simulink model "transfoclarkepark"  (R2018b)
settings: Solver=VariableStepAuto  StartTime=0.0  StopTime=10.0  RelTol=1e-3
settings Model: Creator=lefebvgu  LastModifiedBy=poteaum

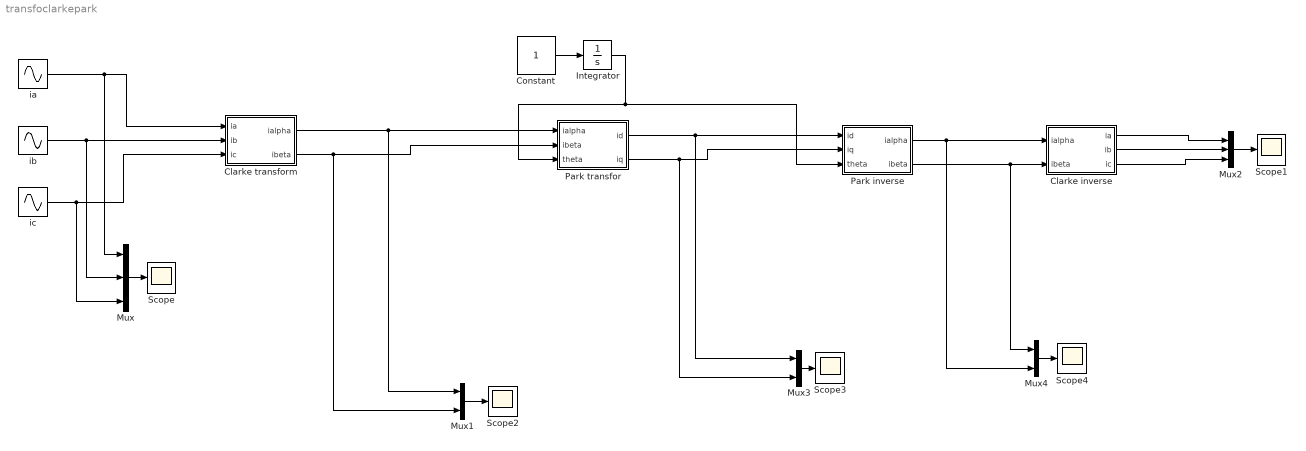
== system transfoclarkepark ==
  Clarke inverse : MATLAB Function  TreatAsAtomicUnit=on
  "Clarke transform " : MATLAB Function  TreatAsAtomicUnit=on
  Constant : Constant  VectorParams1D=off  SampleTime=-1
  Integrator : Integrator
  Mux : Mux  Inputs=3
  Mux1 : Mux  Inputs=2
  Mux2 : Mux  Inputs=3
  Mux3 : Mux  Inputs=2
  Mux4 : Mux  Inputs=2
  "Park inverse " : MATLAB Function  TreatAsAtomicUnit=on
  "Park transfor " : MATLAB Function  TreatAsAtomicUnit=on
  Scope{,1..4} (5 alike) : Scope
  ia : Sin  Amplitude=36  SampleTime=0
  ib : Sin  Amplitude=36  Phase=-2*pi/3  SampleTime=0
  ic : Sin  Amplitude=36  Phase=2*pi/3  SampleTime=0
  wires:
  ia/1 -> Mux/1, "Clarke transform "/1(ia)
  ib/1 -> Mux/2, "Clarke transform "/2(ib)
  ic/1 -> Mux/3, "Clarke transform "/3(ic)
  Mux/1 -> Scope/1
  Clarke inverse/1(ia) -> Mux2/1
  Clarke inverse/2(ib) -> Mux2/2
  Clarke inverse/3(ic) -> Mux2/3
  Mux2/1 -> Scope1/1
  "Clarke transform "/1(ialpha) -> Mux1/1, "Park transfor "/1(ialpha)
  "Clarke transform "/2(ibeta) -> Mux1/2, "Park transfor "/2(ibeta)
  Constant/1 -> Integrator/1
  "Park transfor "/1(id) -> "Park inverse "/1(id), Mux3/1
  "Park transfor "/2(iq) -> Mux3/2, "Park inverse "/2(iq)
  "Park inverse "/1(ialpha) -> Mux4/2, Clarke inverse/1(ialpha)
  "Park inverse "/2(ibeta) -> Mux4/1, Clarke inverse/2(ibeta)
  Mux1/1 -> Scope2/1
  Mux3/1 -> Scope3/1
  Mux4/1 -> Scope4/1
  Integrator/1 -> "Park inverse "/3(theta), "Park transfor "/3(theta)

== matlab function transfoclarkepark/Clarke inverse ==
  data: ialpha input; ia output; ibeta input; ib output; ic output
function [ia,ib,ic]= fcn(ialpha,ibeta)
I = [ialpha; ibeta; 0];
M_C=[1 0 0;1/sqrt(3) 2/sqrt(3) 0; 1 1 1];
solu=inv(M_C)*I;
ia = solu(1);
ib=solu(2);
ic= solu(3);
end

== matlab function transfoclarkepark/Clarke transform  ==
  data: ia input; ialpha output; ib input; ic input; ibeta output
function [ialpha,ibeta]= fcn(ia,ib,ic)
I =[ ia;ib;ic];
M_C=[1 0 0;1/sqrt(3) 2/sqrt(3) 0; 1 1 1];
solu=(M_C)*I;
ialpha= solu(1);
ibeta=solu(2);
end

== matlab function transfoclarkepark/Park transfor  ==
  data: ialpha input; id output; ibeta input; iq output; theta input
function [id,iq]= fcn(ialpha,ibeta,theta)

I=[ialpha;ibeta];
M_P=[cos(theta) sin(theta); -sin(theta) cos(theta)];
solu=M_P*I;
id=solu(1);
iq=solu(2);

end

== matlab function transfoclarkepark/Park inverse  ==
  data: id input; ialpha output; iq input; ibeta output; theta input
function [ialpha,ibeta]= fcn(id,iq,theta)
I=[id; iq]
M_P=[cos(theta) sin(theta); -sin(theta) cos(theta)];
solu=inv(M_P)*I;
ialpha = solu(1);
ibeta=solu(2);
end
